simulink model "main"  (R2021b)
settings: Solver=VariableStepAuto  StartTime=0.0  StopTime=60  RelTol=1e-3
undefined symbols (not defined in the file or in its folder): B, D_LIN, D_QUAD, I0, m, M_A, r_b_b, r_g_b, W
libraries: aerolibguid x1, slpidlib x1
settings Model: Creator=User  LastModifiedBy=saigon
settings SolverCC: AlgebraicLoopSolver=TrustRegion
settings OptimizationCC: LifeSpan=inf
settings DebuggingCC: SFExecutionAtInitializationDiag=none  SFMachineParentedDataDiag=warning  ArithmeticOperatorsInVariantConditions=warning
settings SFSimCC: CustomCodeUndefinedFunction=UseInterfaceOnly
settings CodeAppCC: StateflowObjectComments=on

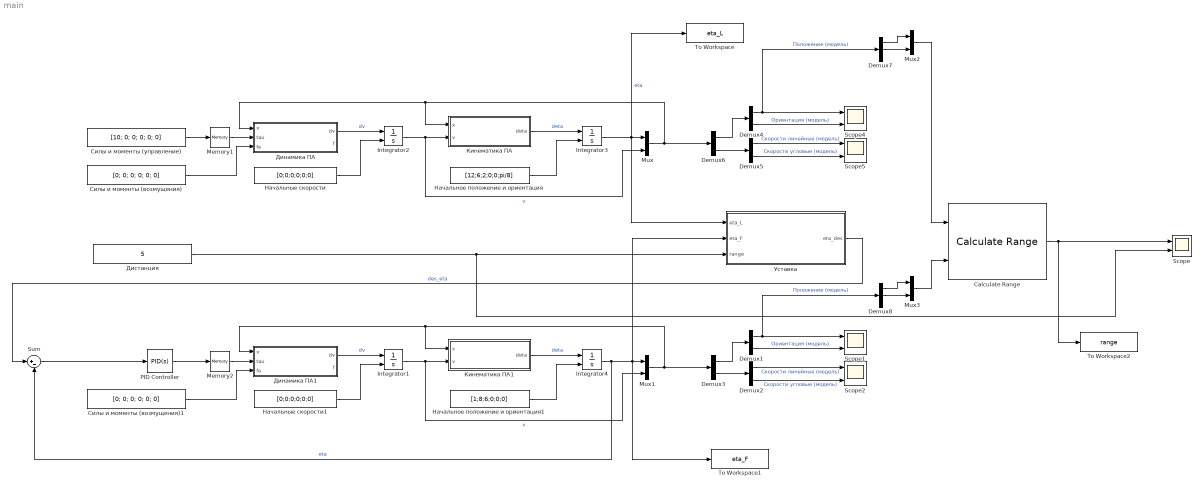
== system main ==
  Calculate Range : aerolibguid/Calculate Range
      settings: SourceProductBaseCode=AE
  Demux{1..6} (6 alike) : Demux  Outputs=2
  Demux7 : Demux  Outputs=3
  Demux8 : Demux  Outputs=3
  Integrator{1..4} (4 alike) : Integrator  InitialConditionSource=external  UpperSaturationLimit=1000  LowerSaturationLimit=-1000
  Memory1 : Memory
  Memory2 : Memory
  Mux{,1..3} (4 alike) : Mux  Inputs=2
  PID Controller : slpidlib/PID Controller  Controller=PID  Form=Parallel  TimeDomain=Continuous-time  UseExternalTs=off  SampleTime=-1  IntegratorMethod=Forward Euler  FilterMethod=Forward Euler  ControllerParametersSource=internal  P=[30;50;150;100;100;50]  I=[30;30;0;50;50;0]  D=[15;15;30;30;30;15]  UseFilter=on  N=100  TunerSelectOption=Transfer Function Based (PID Tuner App)  InitialConditionSource=internal  InitialConditionForIntegrator=0  InitialConditionForFilter=0  DifferentiatorICPrevScaledInput=0  ExternalReset=none  TrackingMode=off  Kt=1  LimitOutput=off  SatLimitsSource=internal  UpperSaturationLimit=inf  LowerSaturationLimit=-inf  LinearizeAsGain=on  AntiWindupMode=none  Kb=1  POutMin=[]  POutMax=[]  IOutMin=[]  IOutMax=[]  DOutMin=[]  DOutMax=[]  NOutMin=[]  NOutMax=[]  SumOutMin=[]  SumOutMax=[]  SaturationOutMin=[]  SaturationOutMax=[]  PParamMin=[]  PParamMax=[]  IParamMin=[]  IParamMax=[]  DParamMin=[]  DParamMax=[]  NParamMin=[]  NParamMax=[]  KbParamMin=[]  KbParamMax=[]  KtParamMin=[]  KtParamMax=[]  KbOutMin=[]  KbOutMax=[]  KtOutMin=[]  KtOutMax=[]  IntegratorOutMin=[]  IntegratorOutMax=[]  FilterOutMin=[]  FilterOutMax=[]  SumI1OutMin=[]  SumI1OutMax=[]  SumI2OutMin=[]  SumI2OutMax=[]  SumI3OutMin=[]  SumI3OutMax=[]  SumI4OutMin=[]  SumI4OutMax=[]  SumDOutMin=[]  SumDOutMax=[]  DifferentiatorOutMin=[]  DifferentiatorOutMax=[]  FilterDiffOutCoefMin=[]  FilterDiffOutCoefMax=[]  ReciprocalOutMin=[]  ReciprocalOutMax=[]  SumDenOutMin=[]  SumDenOutMax=[]  SumNumOutMin=[]  SumNumOutMax=[]  DivideOutMin=[]  DivideOutMax=[]  UdiffTsProdOutMin=[]  UdiffTsProdOutMax=[]  NTsProdOutMin=[]  NTsProdOutMax=[]  UintegralTsProdOutMin=[]  UintegralTsProdOutMax=[]  UngainTsProdOutMin=[]  UngainTsProdOutMax=[]  IntegratorContinuousStateAttributes=''  IntegratorStateMustResolveToSignalObject=off  IntegratorRTWStateStorageClass=Auto  FilterContinuousStateAttributes=''  FilterStateMustResolveToSignalObject=off  FilterRTWStateStorageClass=Auto  ParallelPVariant=InternalParameters  IdealPVariant=Disabled  IVariant=InternalParameters  DVariant=InternalParameters  IntegratorVariant=Continuous  SatVariant=Disabled  AWVariant=Passthrough  PCopyVariant=Disabled  TRVariant=Disabled  FdbkBlocksVariant=Forward  IdealPFdbkVariant=Disabled  SatFdbkVariant=Disabled  DerivativeFilterVariant=ContFilter  NVariant=InternalParameters  NCopyVariant=Disabled  FilterICVariant=InternalICsFilter  IntegratorICVariant=InternalICs  ExternalResetVariant=Disabled  TRSumVariant=Passthrough  SumFdbkVariant=Disabled  SumVariant=Sum_PID  TsampFilterVariant=InternalTs  TsampNgainVariant=Passthrough  TsampIntegralVariant=Passthrough  ExternalSaturationOutDataTypeStr=Inherit: Same as second input
  Scope{,1..2,4..5} (5 alike) : Scope  NumInputPorts=2
  Sum : Sum  Inputs=|+-
  To Workspace : ToWorkspace  VariableName=eta_L  SampleTime=-1
      settings: Save2DSignal=2-D array (concatenate along first dimension)
  To Workspace1 : ToWorkspace  VariableName=eta_F  SampleTime=-1
      settings: Save2DSignal=2-D array (concatenate along first dimension)
  To Workspace2 : ToWorkspace  VariableName=range  SampleTime=-1
      settings: Save2DSignal=2-D array (concatenate along first dimension)
  Динамика ПА : MATLAB Function  TreatAsAtomicUnit=on
  Динамика ПА1 : MATLAB Function  TreatAsAtomicUnit=on
  Дистанция : Constant  Value=5
  Кинематика ПА : MATLAB Function  TreatAsAtomicUnit=on
  Кинематика ПА1 : MATLAB Function  TreatAsAtomicUnit=on
  Начальное положение и ориентация : Constant  Value=[12;6;2;0;0;pi/8]
  Начальное положение и ориентация1 : Constant  Value=[1;8;6;0;0;0]
  Начальные скорости : Constant  Value=[0;0;0;0;0;0]
  Начальные скорости1 : Constant  Value=[0;0;0;0;0;0]
  Силы и моменты (возмущения) : Constant  Value=[0; 0; 0; 0; 0; 0]
  Силы и моменты (возмущения)1 : Constant  Value=[0; 0; 0; 0; 0; 0]
  Силы и моменты (управление) : Constant  Value=[10; 0; 0; 0; 0; 0]
  Уставка : MATLAB Function  TreatAsAtomicUnit=on
  wires:
  Demux4/1 -> Demux7/1, Scope4/1  "Положение (модель)"
  Demux4/2 -> Scope4/2  "Ориентация (модель)"
  Demux5/2 -> Scope5/2  "Скорости угловые (модель)"
  Demux5/1 -> Scope5/1  "Скорости линейные (модель)"
  Demux6/2 -> Demux5/1
  Demux6/1 -> Demux4/1
  Динамика ПА/1(dv) -> Integrator2/1  "dv"
  Силы и моменты (управление)/1 -> Memory1/1
  Integrator2/1 -> Mux/2, Кинематика ПА/2(v)  "v"
  Кинематика ПА/1(deta) -> Integrator3/1  "deta"
  Integrator3/1 -> To Workspace/1, Уставка/1(eta_L), Mux/1  "eta"
  Mux/1 -> Demux6/1, Динамика ПА/1(x), Кинематика ПА/1(x)
  Начальные скорости/1 -> Integrator2/2
  Начальное положение и ориентация/1 -> Integrator3/2
  Memory1/1 -> Динамика ПА/2(tau)
  Силы и моменты (возмущения)/1 -> Динамика ПА/3(fe)
  Силы и моменты (возмущения)1/1 -> Динамика ПА1/3(fe)
  Memory2/1 -> Динамика ПА1/2(tau)
  Начальное положение и ориентация1/1 -> Integrator4/2
  Начальные скорости1/1 -> Integrator1/2
  Mux1/1 -> Кинематика ПА1/1(x), Динамика ПА1/1(x), Demux3/1
  Integrator4/1 -> Sum/2, To Workspace1/1, Уставка/2(eta_F), Mux1/1  "eta"
  Кинематика ПА1/1(deta) -> Integrator4/1  "deta"
  Integrator1/1 -> Кинематика ПА1/2(v), Mux1/2  "v"
  Динамика ПА1/1(dv) -> Integrator1/1  "dv"
  Demux3/1 -> Demux1/1
  Demux3/2 -> Demux2/1
  Demux2/1 -> Scope2/1  "Скорости линейные (модель)"
  Demux2/2 -> Scope2/2  "Скорости угловые (модель)"
  Demux1/2 -> Scope1/2  "Ориентация (модель)"
  Demux1/1 -> Demux8/1, Scope1/1  "Положение (модель)"
  Demux7/1 -> Mux2/1
  Demux7/2 -> Mux2/2
  Mux2/1 -> Calculate Range/1
  Demux8/2 -> Mux3/2
  Demux8/1 -> Mux3/1
  Mux3/1 -> Calculate Range/2
  Calculate Range/1 -> To Workspace2/1, Scope/1
  Дистанция/1 -> Scope/2, Уставка/3(range)
  Уставка/1(eta_des) -> Sum/1  "des_eta"
  Sum/1 -> PID Controller/1
  PID Controller/1 -> Memory2/1

== matlab function main/Динамика ПА1 ==
  data: x input size=12; tau input size=6; fe input size=6; dv output size=6; I0 parameter; r_g_b parameter; m parameter; r_b_b parameter; M_A parameter; D_LIN parameter; D_QUAD parameter; B parameter; W parameter; f output
function [dv, f] = VehicleDynamics(x, tau, fe, I0, r_g_b, m, r_b_b, M_A, D_LIN, D_QUAD, B, W)
n = 6;
eta = x(1:n); 
v = x(7:end);

%% ВСПОМОГАТЕЛЬНЫЕ ФУНКЦИИ
% преобразование в кососимметричную матрицу
S = @(x)([ 0 -x(3) x(2); x(3) 0 -x(1); -x(2) x(1) 0 ]); 

%% РАСЧЕТ ЯКОБИАНА
J_k_o = @(eta)[ 1  0           -sin(eta(5)); ...
                0  cos(eta(4))  cos(eta(5))*sin(eta(4)); ...
                0 -sin(eta(4))  cos(eta(5))*cos(eta(4)) ];
R_I_B = @(eta)[ cos(eta(6))*cos(eta(5))                                        sin(eta(6))*cos(eta(5))                                       -sin(eta(5)); ...
               -sin(eta(6))*cos(eta(4)) + cos(eta(6))*sin(eta(5))*sin(eta(4))  cos(eta(6))*cos(eta(4)) + sin(eta(6))*sin(eta(5))*sin(eta(4))  sin(eta(4))*cos(eta(5)); ...
                sin(eta(6))*sin(eta(4)) + cos(eta(6))*sin(eta(5))*cos(eta(4)) -cos(eta(6))*sin(eta(4)) + sin(eta(6))*sin(eta(5))*cos(eta(4))  cos(eta(4))*cos(eta(5)) ];
J = @(eta)[ R_I_B(eta) zeros(3); ...
            zeros(3)   J_k_o(eta) ];

%% РАСЧЕТ МАТРИЦЫ M
% расчет M_RB
M_RB = [ m*eye(3) -m*S(r_g_b); m*S(r_g_b) I0 ];
% расчет M
M = M_RB + M_A; 

%% РАСЧЕТ C(v)
% расчет C_RB(v)
%C_RB = @(v)([ zeros(3) -m*S(v(1:3)); -m*S(v(1:3)) -S(diag(I0).*v(4:end)) ]); 
C_RB = @(v)[ zeros(3)                           -m*S(v(1:3))-m*S(S(v(4:end))*r_g_b); ...
            -m*S(v(1:3))-m*S(S(v(4:end))*r_g_b)  m*S(S(v(1:3))*r_g_b)-S(I0*v(4:end)) ];
% расчет C_A(v)
diag_M_A = diag(M_A);
C_A = @(v)([ zeros(3) -S(diag_M_A(1:3).*v(1:3));
    -S(diag_M_A(1:3).*v(1:3)) -S(diag_M_A(4:end).*v(4:end))]);
% расчет C(v)
C = @(v)(C_RB(v) + C_A(v)); 
% M11 = M(1:3,1:3); M12 = M(1:3,4:6); M21 = M(4:6,1:3); M22 = M(4:6,4:6);
% C = @(v)[ zeros(3) -S(M11*v(1:3)+M12*v(4:6)); -S(M11*v(1:3)+M12*v(4:6)) -S(M21*v(1:3)+M22*v(4:6)) ];

%% РАСЧЕТ D(v)
D = @(v)(D_LIN + D_QUAD .* diag(abs(v)));

%% РАСЧЕТ g(n)
x_g = r_g_b(1); y_g = r_g_b(2); z_g = r_g_b(3);
x_b = r_b_b(1); y_b = r_b_b(2); z_b = r_b_b(3);
g = @(eta)[ (W-B)*sin(eta(5)); 
           -(W-B)*cos(eta(5))*sin(eta(4)); 
           -(W-B)*cos(eta(5))*cos(eta(4));
           -(y_g*W-y_b*B)*cos(eta(5))*cos(eta(4)) + ...
              (z_g*W-z_b*B)*cos(eta(5))*sin(eta(4));
            (z_g*W-z_b*B)*sin(eta(5)) + ...
              (x_g*W-x_b*B)*cos(eta(5))*cos(eta(4));
           -(x_g*W-x_b*B)*cos(eta(5))*sin(eta(4)) - ...
              (y_g*W-y_b*B)*sin(eta(5)) ];

dv = -M^-1 * ( C(v)*v + D(v)*v + g(eta) - tau - J(eta)' * fe );
f = M * dv;

== matlab function main/Кинематика ПА1 ==
  data: x input size=12; v input size=6; deta output size=6
function deta = VeicleKinematics(x, v)
n = 6;
eta = x(1:n);

%% РАСЧЕТ ЯКОБИАНА
J_k_o = [ 1  0           -sin(eta(5)); ...
          0  cos(eta(4))  cos(eta(5))*sin(eta(4)); ...
          0 -sin(eta(4))  cos(eta(5))*cos(eta(4)) ];
R_I_B = [ cos(eta(6))*cos(eta(5))                                         sin(eta(6))*cos(eta(5))                                        -sin(eta(5)); ...
         -sin(eta(6))*cos(eta(4)) + cos(eta(6))*sin(eta(5))*sin(eta(4))   cos(eta(6))*cos(eta(4)) + sin(eta(6))*sin(eta(5))*sin(eta(4))   sin(eta(4))*cos(eta(5)); ...
          sin(eta(6))*sin(eta(4)) + cos(eta(6))*sin(eta(5))*cos(eta(4))  -cos(eta(6))*sin(eta(4)) + sin(eta(6))*sin(eta(5))*cos(eta(4))   cos(eta(4))*cos(eta(5))];
J = [ R_I_B    zeros(3); ...
      zeros(3) J_k_o  ];

deta = inv(J) * v;

== matlab function main/Динамика ПА ==
  data: x input size=12; tau input size=6; fe input size=6; dv output size=6; I0 parameter; r_g_b parameter; m parameter; r_b_b parameter; M_A parameter; D_LIN parameter; D_QUAD parameter; B parameter; W parameter; f output
function [dv, f] = VehicleDynamics(x, tau, fe, I0, r_g_b, m, r_b_b, M_A, D_LIN, D_QUAD, B, W)
n = 6;
eta = x(1:n); 
v = x(7:end);

%% ВСПОМОГАТЕЛЬНЫЕ ФУНКЦИИ
% преобразование в кососимметричную матрицу
S = @(x)([ 0 -x(3) x(2); x(3) 0 -x(1); -x(2) x(1) 0 ]); 

%% РАСЧЕТ ЯКОБИАНА
J_k_o = @(eta)[ 1  0           -sin(eta(5)); ...
                0  cos(eta(4))  cos(eta(5))*sin(eta(4)); ...
                0 -sin(eta(4))  cos(eta(5))*cos(eta(4)) ];
R_I_B = @(eta)[ cos(eta(6))*cos(eta(5))                                        sin(eta(6))*cos(eta(5))                                       -sin(eta(5)); ...
               -sin(eta(6))*cos(eta(4)) + cos(eta(6))*sin(eta(5))*sin(eta(4))  cos(eta(6))*cos(eta(4)) + sin(eta(6))*sin(eta(5))*sin(eta(4))  sin(eta(4))*cos(eta(5)); ...
                sin(eta(6))*sin(eta(4)) + cos(eta(6))*sin(eta(5))*cos(eta(4)) -cos(eta(6))*sin(eta(4)) + sin(eta(6))*sin(eta(5))*cos(eta(4))  cos(eta(4))*cos(eta(5)) ];
J = @(eta)[ R_I_B(eta) zeros(3); ...
            zeros(3)   J_k_o(eta) ];

%% РАСЧЕТ МАТРИЦЫ M
% расчет M_RB
M_RB = [ m*eye(3) -m*S(r_g_b); m*S(r_g_b) I0 ];
% расчет M
M = M_RB + M_A; 

%% РАСЧЕТ C(v)
% расчет C_RB(v)
%C_RB = @(v)([ zeros(3) -m*S(v(1:3)); -m*S(v(1:3)) -S(diag(I0).*v(4:end)) ]); 
C_RB = @(v)[ zeros(3)                           -m*S(v(1:3))-m*S(S(v(4:end))*r_g_b); ...
            -m*S(v(1:3))-m*S(S(v(4:end))*r_g_b)  m*S(S(v(1:3))*r_g_b)-S(I0*v(4:end)) ];
% расчет C_A(v)
diag_M_A = diag(M_A);
C_A = @(v)([ zeros(3) -S(diag_M_A(1:3).*v(1:3));
    -S(diag_M_A(1:3).*v(1:3)) -S(diag_M_A(4:end).*v(4:end))]);
% расчет C(v)
C = @(v)(C_RB(v) + C_A(v)); 
% M11 = M(1:3,1:3); M12 = M(1:3,4:6); M21 = M(4:6,1:3); M22 = M(4:6,4:6);
% C = @(v)[ zeros(3) -S(M11*v(1:3)+M12*v(4:6)); -S(M11*v(1:3)+M12*v(4:6)) -S(M21*v(1:3)+M22*v(4:6)) ];

%% РАСЧЕТ D(v)
D = @(v)(D_LIN + D_QUAD .* diag(abs(v)));

%% РАСЧЕТ g(n)
x_g = r_g_b(1); y_g = r_g_b(2); z_g = r_g_b(3);
x_b = r_b_b(1); y_b = r_b_b(2); z_b = r_b_b(3);
g = @(eta)[ (W-B)*sin(eta(5)); 
           -(W-B)*cos(eta(5))*sin(eta(4)); 
           -(W-B)*cos(eta(5))*cos(eta(4));
           -(y_g*W-y_b*B)*cos(eta(5))*cos(eta(4)) + ...
              (z_g*W-z_b*B)*cos(eta(5))*sin(eta(4));
            (z_g*W-z_b*B)*sin(eta(5)) + ...
              (x_g*W-x_b*B)*cos(eta(5))*cos(eta(4));
           -(x_g*W-x_b*B)*cos(eta(5))*sin(eta(4)) - ...
              (y_g*W-y_b*B)*sin(eta(5)) ];

dv = -M^-1 * ( C(v)*v + D(v)*v + g(eta) - tau - J(eta)' * fe );
f = M * dv;

== matlab function main/Уставка ==
  data: eta_L input size=6; eta_F input size=6; eta_des output size=6; range input size=1
function eta_des = DesiredETA(eta_L, eta_F, range)
x1 = eta_L(1) + (range * (eta_F(1) - eta_L(1))) / sqrt( (eta_F(1) - eta_L(1))^2 + (eta_F(2) - eta_L(2))^2 );
x2 = eta_L(1) - (range * (eta_F(1) - eta_L(1))) / sqrt( (eta_F(1) - eta_L(1))^2 + (eta_F(2) - eta_L(2))^2 );

y1 = eta_L(2) + (range * (eta_F(1) - eta_L(1))) / sqrt( (eta_F(1) - eta_L(1))^2 + (eta_F(2) - eta_L(2))^2 );
y2 = eta_L(2) - (range * (eta_F(1) - eta_L(1))) / sqrt( (eta_F(1) - eta_L(1))^2 + (eta_F(2) - eta_L(2))^2 );

dist1 = sqrt((x1 - eta_F(1))^2 + (y1 - eta_F(2))^2);
dist2 = sqrt((x2 - eta_F(1))^2 + (y2 - eta_F(2))^2);

[~, idx] = min([dist1 dist2]);

if idx == 1
    x = x1;
    y = y1;
else
    x = x2;
    y = y2;
end

eta_des = [ x; y; eta_L(3); 0; 0; eta_L(6) - eta_F(6) ];

== matlab function main/Кинематика ПА ==
  data: x input size=12; v input size=6; deta output size=6
function deta = VeicleKinematics(x, v)
n = 6;
eta = x(1:n);

%% РАСЧЕТ ЯКОБИАНА
J_k_o = [ 1  0           -sin(eta(5)); ...
          0  cos(eta(4))  cos(eta(5))*sin(eta(4)); ...
          0 -sin(eta(4))  cos(eta(5))*cos(eta(4)) ];
R_I_B = [ cos(eta(6))*cos(eta(5))                                         sin(eta(6))*cos(eta(5))                                        -sin(eta(5)); ...
         -sin(eta(6))*cos(eta(4)) + cos(eta(6))*sin(eta(5))*sin(eta(4))   cos(eta(6))*cos(eta(4)) + sin(eta(6))*sin(eta(5))*sin(eta(4))   sin(eta(4))*cos(eta(5)); ...
          sin(eta(6))*sin(eta(4)) + cos(eta(6))*sin(eta(5))*cos(eta(4))  -cos(eta(6))*sin(eta(4)) + sin(eta(6))*sin(eta(5))*cos(eta(4))   cos(eta(4))*cos(eta(5))];
J = [ R_I_B    zeros(3); ...
      zeros(3) J_k_o  ];

deta = inv(J) * v;
